simulink model "evitar_choque2023v"  (R2023b)
settings: Solver=VariableStepAuto  StartTime=0.0  StopTime=10.0  RelTol=1e-3
libraries: simulink x2
settings Model: Creator=Usuario_UMA  LastModifiedBy=julia

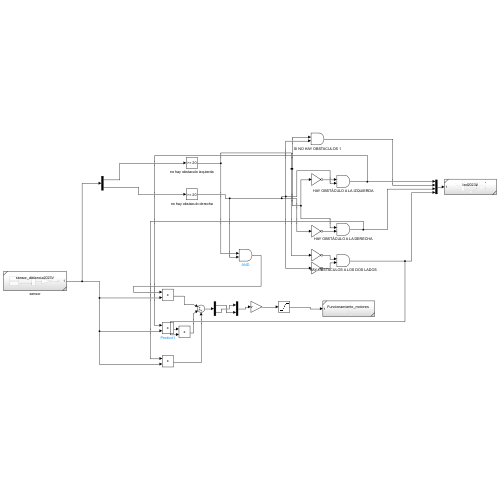
[thumbnail: Simulink's stored preview of the top-level diagram]
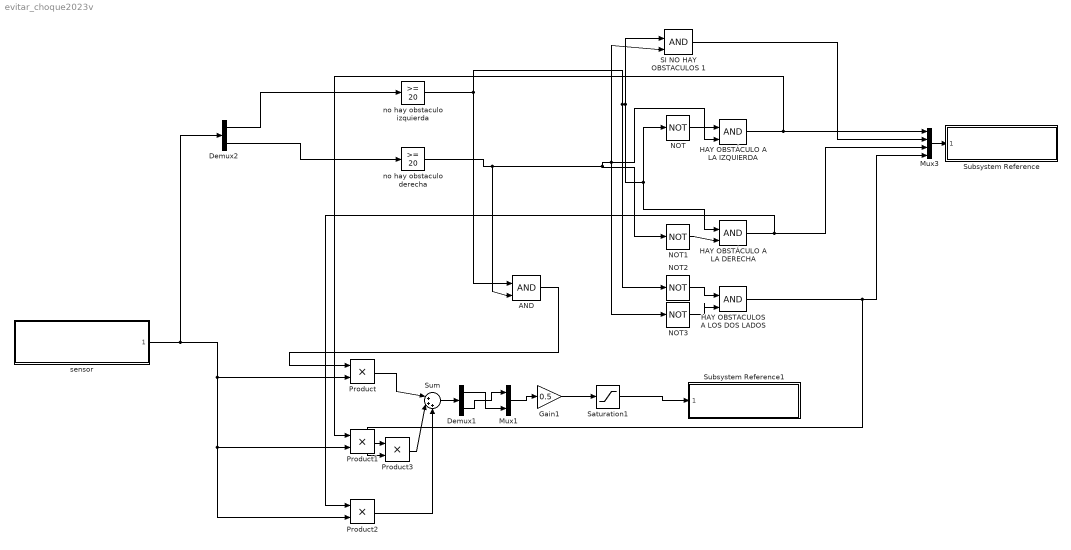
== system evitar_choque2023v ==
  AND : Logic  IconShape=distinctive  AllPortsSameDT=off  OutDataTypeStr=boolean
  Demux1 : Demux  Outputs=2
  Demux2 : Demux  Outputs=2
  Gain1 : Gain  Gain=0.5
  HAY OBSTACULOS A LOS DOS LADOS : Logic  IconShape=distinctive  AllPortsSameDT=off  OutDataTypeStr=boolean
  HAY OBSTÁCULO A LA DERECHA : Logic  IconShape=distinctive  AllPortsSameDT=off  OutDataTypeStr=boolean
  HAY OBSTÁCULO A LA IZQUIERDA : Logic  IconShape=distinctive  AllPortsSameDT=off  OutDataTypeStr=boolean
  Mux1 : Mux  Inputs=2
  Mux3 : Mux
  NOT{,1..3} (4 alike) : Logic  Operator=NOT  IconShape=distinctive  AllPortsSameDT=off  OutDataTypeStr=boolean
  Product{,1..3} (4 alike) : Product
  SI NO HAY OBSTACULOS 1 : Logic  IconShape=distinctive  AllPortsSameDT=off  OutDataTypeStr=boolean
  Saturation1 : Saturate
  Subsystem Reference : Subsystem  ReferencedSubsystem=led2023V
  Subsystem Reference1 : Subsystem  ReferencedSubsystem=Funcionamiento_motores
  Sum : Sum  Inputs=|+++
  no hay obstaculo derecha : simulink/Logic and Bit Operations/Compare To Constant  relop=>=  const=20  OutDataTypeStr=boolean
  no hay obstaculo izquierda : simulink/Logic and Bit Operations/Compare To Constant  relop=>=  const=20  OutDataTypeStr=boolean
  sensor : Subsystem  ReferencedSubsystem=sensor_distancia2023V
  wires:
  NOT1/1 -> HAY OBSTÁCULO A LA DERECHA/2
  sensor/1 -> Product2/2, Product1/2, Product/2, Demux2/1
  no hay obstaculo derecha/1 -> AND/2, HAY OBSTÁCULO A LA IZQUIERDA/2, SI NO HAY OBSTACULOS 1/2, NOT3/1, NOT1/1
  no hay obstaculo izquierda/1 -> AND/1, NOT2/1, SI NO HAY OBSTACULOS 1/1, HAY OBSTÁCULO A LA DERECHA/1, NOT/1
  SI NO HAY OBSTACULOS 1/1 -> Mux3/2
  AND/1 -> Product/1
  Demux2/1 -> no hay obstaculo izquierda/1
  NOT3/1 -> HAY OBSTACULOS A LOS DOS LADOS/2
  HAY OBSTÁCULO A LA IZQUIERDA/1 -> Product1/1, Mux3/1
  NOT/1 -> HAY OBSTÁCULO A LA IZQUIERDA/1
  HAY OBSTÁCULO A LA DERECHA/1 -> Product2/1, Mux3/3
  NOT2/1 -> HAY OBSTACULOS A LOS DOS LADOS/1
  Demux2/2 -> no hay obstaculo derecha/1
  Saturation1/1 -> Subsystem Reference1/1
  HAY OBSTACULOS A LOS DOS LADOS/1 -> Product3/2, Mux3/4
  Demux1/1 -> Mux1/2
  Gain1/1 -> Saturation1/1
  Mux1/1 -> Gain1/1
  Demux1/2 -> Mux1/1
  Mux3/1 -> Subsystem Reference/1
  Product/1 -> Sum/1
  Sum/1 -> Demux1/1
  Product1/1 -> Product3/1
  Product3/1 -> Sum/2
  Product2/1 -> Sum/3
